simulink model "Three_ph_T_YDparam2"  (R2024b)
settings: Solver=VariableStepAuto  StartTime=0.0  StopTime=10  RelTol=1e-3
values from neighbouring files (symbols this model uses):
  Lp = 0    [Three_ph_TFimptest_Y_D_vFinal.m]
  Ls = 0.084225    [Three_ph_TFimptest_Y_D_vFinal.m]
  P = 200e6    (= 200000000)    [Three_ph_TFimptest_Y_D_vFinal.m]
  Rp = 4.3218    [Three_ph_TFimptest_Y_D_vFinal.m]
  Rs = 0.7938    [Three_ph_TFimptest_Y_D_vFinal.m]
  V = 20e3    (= 20000)    [Three_ph_TFimptest_Y_D_vFinal.m]
  V1 = 2 * V2    (= 20000)    [Three_ph_TFimptest_Y_D_vFinal.m]
  V2 = 1e4    (= 10000)    [Three_ph_TFimptest_Y_D_vFinal.m]
undefined symbols (not defined in the file or in its folder): D1, Delta
libraries: spsGroundLib x3, spsThreePhaseTransformerTwoWindingsLib x2, spsThreePhaseVIMeasurementLib x2, spsThreePhaseProgrammableVoltageSourceLib x1, sps_lib x1
settings Model: PacingRate=0.110000  Creator=salsarayreh  LastModifiedBy=PC1

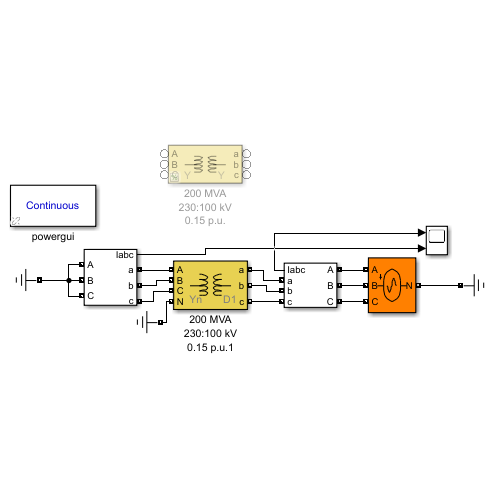
[thumbnail: Simulink's stored preview of the top-level diagram]
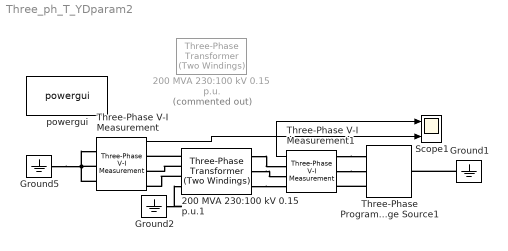
== system Three_ph_T_YDparam2 ==
  200 MVA 230:100 kV 0.15 p.u. : spsThreePhaseTransformerTwoWindingsLib/Three-Phase Transformer (Two Windings)  Commented=on  Winding1Connection=Y  Winding2Connection=Y  CoreType=Three single-phase transformers  SetSaturation=off  Hysteresis=off  DataFile='hysteresis'  SetInitialFlux=off  Measurements=None  UNITS=SI  NominalPower=[200e6 , 50]  Winding1=[2.1045e+05 0.55362 0.052866]  Winding2=[1e+05 0.125 0.011937]  Rm=1.1072e+05  Lm=352.44  L0=0.5  Saturation=[0 0;9.3114 683.7;785.26 875.13]  InitialFluxes=[-1.03850588171453 0.527233233676132 0.511272648041703]  BreakLoop=off  DiscreteSolver=Trapezoidal iterative  DataType=on  TransfoNumber=0
  200 MVA 230:100 kV 0.15 p.u.1 : spsThreePhaseTransformerTwoWindingsLib/Three-Phase Transformer (Two Windings)  Winding1Connection=Yn  Winding2Connection=Delta (D1)  CoreType=Three single-phase transformers  SetSaturation=off  Hysteresis=off  DataFile='hysteresis'  SetInitialFlux=off  Measurements=None  UNITS=SI  NominalPower=[P , 50]  Winding1="[ V1 Rp  Lp ]"  Winding2="[ V2 Rs  Ls  ]"  Rm=Rm  Lm=Lm  L0=0.5  Saturation=[0 0;9.3114 683.7;785.26 875.13]  InitialFluxes=[-1.03850588171453 0.527233233676132 0.511272648041703]  BreakLoop=off  DiscreteSolver=Trapezoidal iterative  DataType=on  TransfoNumber=0
  Ground1 : spsGroundLib/Ground  LConnTagsString=a
  Ground2 : spsGroundLib/Ground  LConnTagsString=a
  Ground5 : spsGroundLib/Ground  LConnTagsString=a
  Scope1 : Scope  NumInputPorts=2
  Three-Phase Programmable Voltage Source1 : spsThreePhaseProgrammableVoltageSourceLib/Three-Phase Programmable Voltage Source  PositiveSequence="[V  0  50]"  VariationEntity=Amplitude  VariationType=Step  VariationTypeAlt=Step  VariationStep=-0.1  VariationRate=10  VariationMagnitude=0.3  VariationFrequency=2  VariationTiming="[0  0.14] + 1.5"  VariationPhaseA=off  Amplitudes=[1 0.8 1.2 1.0]  TimeValues=[0 0.1 0.15 0.2]  HarmonicGeneration=off  HarmonicA="[2 0.10  0  2]"  HarmonicB="[2  0  35 2]"  Timing="[1.2  99]"  BusType=swing  Pref=0  Qref=0  Qmin=-inf  Qmax=inf
  Three-Phase V-I Measurement : spsThreePhaseVIMeasurementLib/Three-Phase V-I Measurement  VoltageMeasurement=no  SetLabelV=off  LabelV=Vabc  Vpu=off  VpuLL=off  CurrentMeasurement=yes  SetLabelI=off  LabelI=Iabc  Ipu=off  Pbase=100e6  Vbase=500e3  OutputType=Complex  PhasorSimulation=off  PSBequivalent=0
  Three-Phase V-I Measurement1 : spsThreePhaseVIMeasurementLib/Three-Phase V-I Measurement  VoltageMeasurement=no  SetLabelV=off  LabelV=Vabc  Vpu=off  VpuLL=off  CurrentMeasurement=yes  SetLabelI=off  LabelI=Iabc  Ipu=off  Pbase=100e6  Vbase=500e3  OutputType=Complex  PhasorSimulation=off  PSBequivalent=0
  powergui : sps_lib/powergui  Priority=1  SimulationMode=Continuous  SampleTime=50e-6  frequency=60  Iterations=50  frequencyindice=50  Pbase=100e6  ErrMax=1e-4  UnitsV=kV  UnitsW=MW  buscounter=0  FunctionMessages=off  echomessages=off  EnableUseOfTLC=off  CurrentSourceSwitches=off  DisableSnubberDevices=off  DisableRonSwitches=off  DisableVfSwitches=off  DisplayEquations=off  AutomaticDiscreteSolvers=off  SolverType=Tustin/Backward Euler (TBE)  Interpol=off  ExternalGateDelay=off  methode=off  Ts=100  x0status=blocks  SPID=on  SwTol=0  HookPort=off  NonlinearTolerance=1e-4  nMaxIteration=100  ContinueOnMaxIteration=off  RestoreLinks=warning  ResistiveCurrentMeasurement=off  Frange=[0:2:500]  Ylog=off  Xlog=on  ShowGrid=off  save=off  variable=ZData  structure=0  ZoomFFT=off  StartTime=0.0  cycles=1  DisplayStyle=1  fundamental=60  FreqAxis=off  MaxFrequency=1000  frequencyindicesteady=1  RmsSteady=1  display=off
  wires:
  Three-Phase V-I Measurement/1 -> Scope1/2
  Three-Phase V-I Measurement1/1 -> Scope1/1
  connections:
  200 MVA 230:100 kV 0.15 p.u.1/LConn1 -- Three-Phase V-I Measurement/RConn1
  200 MVA 230:100 kV 0.15 p.u.1/LConn3 -- Three-Phase V-I Measurement/RConn3
  200 MVA 230:100 kV 0.15 p.u.1/LConn2 -- Three-Phase V-I Measurement/RConn2
  Ground5/LConn1 -- Three-Phase V-I Measurement/LConn3 -- Three-Phase V-I Measurement/LConn1 -- Three-Phase V-I Measurement/LConn2
  Ground1/LConn1 -- Three-Phase Programmable Voltage Source1/LConn1
  200 MVA 230:100 kV 0.15 p.u.1/RConn3 -- Three-Phase V-I Measurement1/RConn3
  Three-Phase V-I Measurement1/LConn2 -- Three-Phase Programmable Voltage Source1/RConn2
  Three-Phase Programmable Voltage Source1/RConn3 -- Three-Phase V-I Measurement1/LConn3
  Three-Phase V-I Measurement1/LConn1 -- Three-Phase Programmable Voltage Source1/RConn1
  200 MVA 230:100 kV 0.15 p.u.1/RConn2 -- Three-Phase V-I Measurement1/RConn2
  200 MVA 230:100 kV 0.15 p.u.1/RConn1 -- Three-Phase V-I Measurement1/RConn1
  Ground2/LConn1 -- 200 MVA 230:100 kV 0.15 p.u.1/LConn4
